simulink model "LinearniModeliDT"  (R2020b)
settings: Solver=VariableStepAuto  StartTime=0.0  StopTime=140  RelTol=1e-3
undefined symbols (not defined in the file or in its folder): DT5, DT6, Udt5, Udt6
libraries: powerlib_meascontrol x1
settings Model: Creator=Acer  LastModifiedBy=Acer
settings ModelReferenceCC: EnableParallelModelReferenceBuilds=on

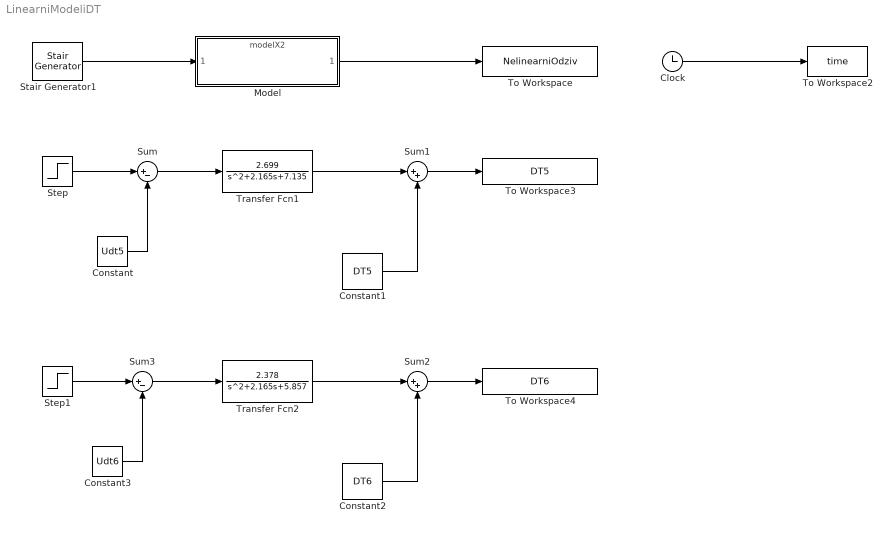
== system LinearniModeliDT ==
  Clock : Clock
  Constant : Constant  Value=Udt5
  Constant1 : Constant  Value=DT5
  Constant2 : Constant  Value=DT6
  Constant3 : Constant  Value=Udt6
  Model : ModelReference  ModelNameDialog=modelX2.slx  SimulationMode=Normal  ModelReferenceVersion=1.9
  Stair Generator1 : powerlib_meascontrol/Pulse & Signal Generators/Stair Generator  t=0:20:100  e=5:0.5:7.5  Ts=0
  Step : Step  Time=20  Before=5  After=5.5  SampleTime=0
  Step1 : Step  Time=60  Before=6  After=6.5  SampleTime=0
  Sum : Sum  Inputs=|+-
  Sum1 : Sum  Inputs=|++
  Sum2 : Sum  Inputs=|++
  Sum3 : Sum  Inputs=|+-
  To Workspace : ToWorkspace  VariableName=NelinearniOdziv  SampleTime=-1
  To Workspace2 : ToWorkspace  VariableName=time  SampleTime=-1
  To Workspace3 : ToWorkspace  VariableName=DT5  SampleTime=-1
  To Workspace4 : ToWorkspace  VariableName=DT6  SampleTime=-1
  Transfer Fcn1 : TransferFcn  Numerator=[2.699]  Denominator=[1 2.165 7.135]
  Transfer Fcn2 : TransferFcn  Numerator=[2.378]  Denominator=[1 2.165 5.857]
  wires:
  Constant1/1 -> Sum1/2
  Transfer Fcn1/1 -> Sum1/1
  Clock/1 -> To Workspace2/1
  Sum2/1 -> To Workspace4/1
  Model/1 -> To Workspace/1
  Sum1/1 -> To Workspace3/1
  Constant2/1 -> Sum2/2
  Stair Generator1/1 -> Model/1
  Transfer Fcn2/1 -> Sum2/1
  Step/1 -> Sum/1
  Sum/1 -> Transfer Fcn1/1
  Constant/1 -> Sum/2
  Constant3/1 -> Sum3/2
  Step1/1 -> Sum3/1
  Sum3/1 -> Transfer Fcn2/1
